simulink model "gm_dut_shape_mod"  (R2020b)
settings: Solver=FixedStepDiscrete  StartTime=0.0  StopTime=10.0  RelTol=1e-3
libraries: commdigbbndpm3 x1, commrandsrc3 x1
settings Model: Creator=wardo  LastModifiedBy=wardo
settings DataIOCC: LimitDataPoints=on  SaveOutput=off  SaveTime=off
settings OptimizationCC: BlockReduction=off  ConditionallyExecuteInputs=off  DefaultParameterBehavior=Inlined  LifeSpan=inf
settings DebuggingCC: AlgebraicLoopMsg=error  InheritedTsInSrcMsg=none  SingleTaskRateTransMsg=error  AllowSymbolicDim=off  StrictBusMsg=ErrorOnBusTreatedAsVector  SFUnexpectedBacktrackingDiag=warning  SFNoUnconditionalDefaultTransitionDiag=warning  SFExecutionAtInitializationDiag=none  ArithmeticOperatorsInVariantConditions=warning
settings HardwareCC: ProdBitPerPointer=32  ProdBitPerSizeT=32  ProdBitPerPtrDiffT=32  ProdLargestAtomicFloat=None  ProdIntDivRoundTo=Undefined  ProdEndianess=Unspecified  ProdWordSize=32  ProdHWDeviceType=ASIC/FPGA->ASIC/FPGA  ProdEqTarget=off
settings SFSimCC: SimUseLocalCustomCode=off  CustomCodeUndefinedFunction=UseInterfaceOnly
settings RTWCC: RTWUseLocalCustomCode=off
settings CodeAppCC: StateflowObjectComments=on
settings GRTTargetCC: TargetLangStandard=C89/C90 (ANSI)
settings ConfigComp: CovScope=ReferencedModels  CovMetricSettings=dw  CovSaveCumulativeToWorkspaceVar=on  CovSaveSingleToWorkspaceVar=on  CovExternalEMLEnable=off  CovSFcnEnable=off

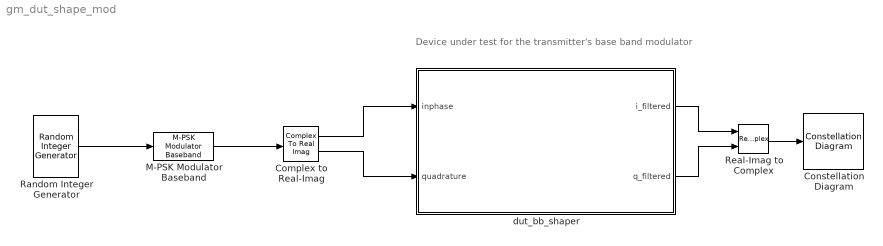
== system gm_dut_shape_mod ==
  note: Device under test for the transmitter's base band modulator
  Complex to Real-Imag : ComplexToRealImag
  Constellation Diagram : ConstellationDiagram
  M-PSK Modulator Baseband : commdigbbndpm3/M-PSK Modulator Baseband  M=8  InType=Bit  Enc=Gray  Mapping=[0:7]  Ph=0  outDtype=Fixed-point  outWordLen=18  outUDDataType=sfix(16)  outFracLenMode=User-defined  outFracLen=14  outDataTypeStr=fixdt(1,18,14)  outLastDataTypeStr=fixdt(1,18,14)
      settings: SourceProductName=Communications Toolbox
  Random Integer Generator : commrandsrc3/Random Integer Generator  SetSize=2  SeedSource=Auto  Seed=0  SampleTime=1  SamplesPerFrame=64800  OutputDataType=double  SimulateUsing=Interpreted execution
  Real-Imag to Complex : RealImagToComplex
  dut_bb_shaper : Subsystem
  wires:
  dut_bb_shaper/2(q_filtered) -> Real-Imag to Complex/2
  dut_bb_shaper/1(i_filtered) -> Real-Imag to Complex/1
  Real-Imag to Complex/1 -> Constellation Diagram/1
  Random Integer Generator/1 -> M-PSK Modulator Baseband/1
  M-PSK Modulator Baseband/1 -> Complex to Real-Imag/1
  Complex to Real-Imag/2 -> dut_bb_shaper/2(quadrature)
  Complex to Real-Imag/1 -> dut_bb_shaper/1(inphase)

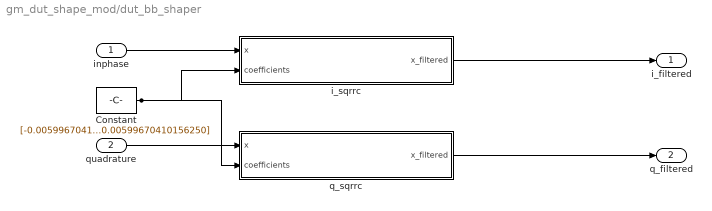
== system gm_dut_shape_mod/dut_bb_shaper ==
  inphase : Inport  OutDataTypeStr=fixdt(1, 18, 14)  PortDimensions=[21600 1]  SampleTime=64800
  quadrature : Inport  Port=2  OutDataTypeStr=fixdt(1, 18, 14)  PortDimensions=[21600 1]  SampleTime=64800
  Constant : Constant  Value=[-0.00599670410156250,-0.00514221191406250,-0.00289916992187500,0.000442504882812500,0.00431823730468750,0.00794982910156250,0.0104980468750000,0.0112304687500000,0.00967407226562500,0.00578308105468750,0,-0.00680541992187500,-0.0134124755859375,-0.0184326171875000,-0.0205841064453125,-0.0189819335937500,-0.0133361816406250,-0.00410461425781250,0.00752258300781250,0.0196380615234375,0.0300140380859375,0.0363464355468750,0.0367584228515625,0.0301208496093750,0.0164794921875000,-0.00291442871093750,-0.0254821777343750,-0.0476837158203125,-0.0653228759765625,-0.0742187500000000,-0.0707244873046875,-0.0524291992187500,-0.0185852050781250,0.0296783447265625,0.0892028808593750,0.155227661132813,0.221755981445313,0.282333374023438,0.330810546875000,0.362121582031250,0.372940063476563,0.362121582031250,0.330810546875000,0.282333374023438,0.221755981445313,0.155227661132813,0.0892028808593750,0.0296783447265625,-0.0185852050781250,-0.0524291992187500,-0.0707244873046875,-0.0742187500000000,-0.0653228759765625,-0.0476837158203125,-0.0254821777343750,-0.00291442871093750,0.0164794921875000,0.0301208496093750,0.0367584228515625,0.0363464355468750,0.0300140380859375,0.0196380615234375,0.00752258300781250,-0.00410461425781250,-0.0133361816406250,-0.0189819335937500,-0.0205841064453125,-0.0184326171875000,-0.0134124755859375,-0.00680541992187500,0,0.00578308105468750,0.00967407226562500,0.0112304687500000,0.0104980468750000,0.00794982910156250,0.00431823730468750,0.000442504882812500,-0.00289916992187500,-0.00514221191406250,-0.00599670410156250]  OutDataTypeStr=fixdt(1,16)  SampleTime=-1
  i_sqrrc : Subsystem
  q_sqrrc : Subsystem
  i_filtered : Outport  VectorParamsAs1DForOutWhenUnconnected=off
  q_filtered : Outport  Port=2  VectorParamsAs1DForOutWhenUnconnected=off
  wires:
  inphase/1 -> i_sqrrc/1(x)
  quadrature/1 -> q_sqrrc/1(x)
  Constant/1 -> q_sqrrc/2(coefficients), i_sqrrc/2(coefficients)
  i_sqrrc/1(x_filtered) -> i_filtered/1
  q_sqrrc/1(x_filtered) -> q_filtered/1

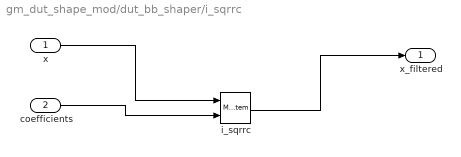
== system gm_dut_shape_mod/dut_bb_shaper/i_sqrrc ==
  x : Inport  OutDataTypeStr=fixdt(1, 18, 14)  PortDimensions=[21600 1]  SampleTime=64800
  coefficients : Inport  Port=2  OutDataTypeStr=fixdt(1, 16, 16)  PortDimensions=[81]  SampleTime=64800
  i_sqrrc : MATLABSystem  System=transmit_srrc_filter  l=21600  interpolation_factor=8  SimulateUsing=Code generation
      mask Type: transmit_srrc_filter
      mask Display:
      | disp('transmit_srrc_filter');
      | port_label('input',1,'x');
      | port_label('input',2,'coefficients');
      | port_label('output',1,'x_filtered');
  x_filtered : Outport
  wires:
  x/1 -> i_sqrrc/1
  coefficients/1 -> i_sqrrc/2
  i_sqrrc/1 -> x_filtered/1

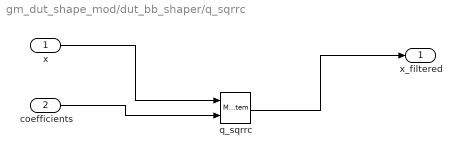
== system gm_dut_shape_mod/dut_bb_shaper/q_sqrrc ==
  x : Inport  OutDataTypeStr=fixdt(1, 18, 14)  PortDimensions=[21600 1]  SampleTime=64800
  coefficients : Inport  Port=2  OutDataTypeStr=fixdt(1, 16, 16)  PortDimensions=[81]  SampleTime=64800
  q_sqrrc : MATLABSystem  System=transmit_srrc_filter  l=21600  interpolation_factor=8  SimulateUsing=Code generation
      mask Type: transmit_srrc_filter
      mask Display:
      | disp('transmit_srrc_filter');
      | port_label('input',1,'x');
      | port_label('input',2,'coefficients');
      | port_label('output',1,'x_filtered');
  x_filtered : Outport
  wires:
  x/1 -> q_sqrrc/1
  coefficients/1 -> q_sqrrc/2
  q_sqrrc/1 -> x_filtered/1
